simulink model "problem_02_sim"  (R2020a)
settings: Solver=VariableStepAuto  StartTime=0.0  StopTime=10.0  RelTol=1e-3
values from neighbouring files (symbols this model uses):
  delta_a = 0    [problem_02.m]
  delta_y = 0    [problem_02.m]
  rho = 1    [problem_02.m]
libraries: cstblocks x2
settings Model: Creator=davidearcolini  LastModifiedBy=davidearcolini

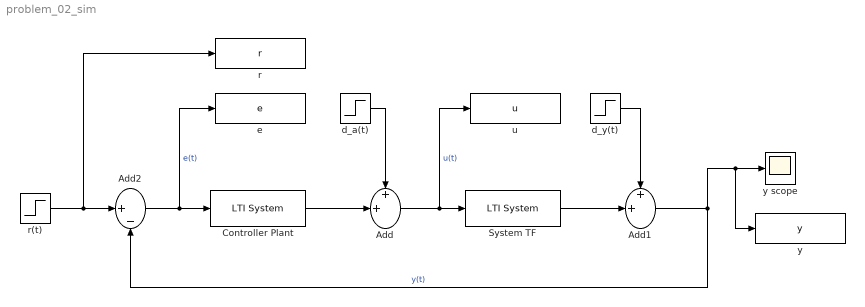
== system problem_02_sim ==
  Add : Sum  Inputs=++|
  Add1 : Sum  Inputs=++|
  Add2 : Sum  Inputs=|+-
  Controller Plant : cstblocks/LTI System  sys=C  IC=[]
  System TF : cstblocks/LTI System  sys=G  IC=[]
  d_a(t) : Step  Time=0  After=delta_a  SampleTime=0
  d_y(t) : Step  Time=0  After=delta_y  SampleTime=0
  e : ToWorkspace  VariableName=e  SaveFormat=Timeseries  SampleTime=-1
  r : ToWorkspace  VariableName=r  SaveFormat=Timeseries  SampleTime=-1
  r(t) : Step  Time=0  After=rho  SampleTime=0
  u : ToWorkspace  VariableName=u  SaveFormat=Timeseries  SampleTime=-1
  y : ToWorkspace  VariableName=y  SaveFormat=Timeseries  SampleTime=-1
  y scope : Scope
  wires:
  Controller Plant/1 -> Add/2
  Add/1 -> u/1, System TF/1  "u(t)"
  d_a(t)/1 -> Add/1
  System TF/1 -> Add1/2
  d_y(t)/1 -> Add1/1
  Add1/1 -> y/1, y scope/1, Add2/2  "y(t)"
  Add2/1 -> e/1, Controller Plant/1  "e(t)"
  r(t)/1 -> r/1, Add2/1
